simulink model "KaplunenkoDD_Task2"  (R2020a)
settings: Solver=VariableStepAuto  StartTime=0.0  StopTime=100  RelTol=1e-3  EnableMultiTasking=on
libraries: simulink x2
settings Model: Creator=Boris  LastModifiedBy=Dmitry Kaplunenko
settings DataIOCC: SaveOutput=off  SignalLogging=off  DSMLogging=off  SaveTime=off  ReturnWorkspaceOutputs=off
settings OptimizationCC: LifeSpan=inf
settings DebuggingCC: SFUnexpectedBacktrackingDiag=warning  SFNoUnconditionalDefaultTransitionDiag=warning  SFExecutionAtInitializationDiag=none  ArithmeticOperatorsInVariantConditions=warning
settings SFSimCC: SimUseLocalCustomCode=off  CustomCodeUndefinedFunction=UseInterfaceOnly
settings RTWCC: RTWUseLocalCustomCode=off
settings CodeAppCC: StateflowObjectComments=on
settings GRTTargetCC: TargetLangStandard=C89/C90 (ANSI)
settings ConfigComp: CovMetricSettings=dw  CovHtmlReporting=on  CovSaveCumulativeToWorkspaceVar=on  CovSaveSingleToWorkspaceVar=on  CovExternalEMLEnable=off

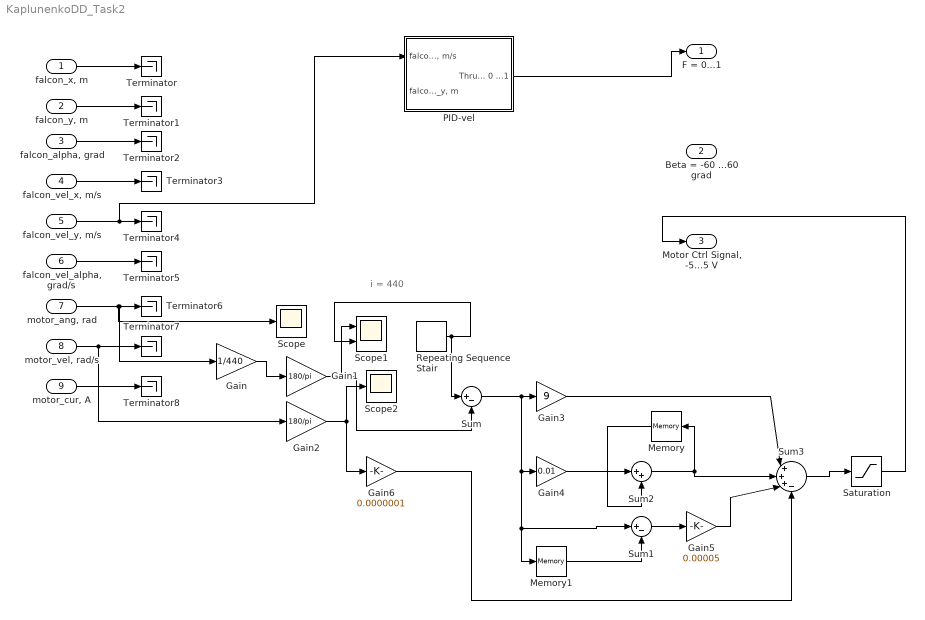
== system KaplunenkoDD_Task2 ==
  note: i = 440
  "falcon_x, m" : Inport  OutDataTypeStr=double  PortDimensions=1  SampleTime=[0.01,0]
  "falcon_y, m" : Inport  Port=2  OutDataTypeStr=double  PortDimensions=1  SampleTime=[0.01,0]
  "falcon_alpha, grad" : Inport  Port=3  OutDataTypeStr=double  PortDimensions=1  SampleTime=[0.01,0]
  "falcon_vel_x, m/s" : Inport  Port=4  OutDataTypeStr=double  PortDimensions=1  SampleTime=[0.01,0]
  "falcon_vel_y, m/s" : Inport  Port=5  OutDataTypeStr=double  PortDimensions=1  SampleTime=[0.01,0]
  "falcon_vel_alpha, grad/s" : Inport  Port=6  OutDataTypeStr=double  PortDimensions=1  SampleTime=[0.01,0]
  "motor_ang, rad" : Inport  Port=7  OutDataTypeStr=double  PortDimensions=1  SampleTime=[0.01,0]
  "motor_vel, rad/s" : Inport  Port=8  OutDataTypeStr=double  PortDimensions=1  SampleTime=[0.01,0]
  "motor_cur, A" : Inport  Port=9  OutDataTypeStr=double  PortDimensions=1  SampleTime=[0.01,0]
  Gain : Gain  Gain=1/440
  Gain1 : Gain  Gain=180/pi
  Gain2 : Gain  Gain=180/pi
  Gain3 : Gain  Gain=9
  Gain4 : Gain  Gain=0.01
  Gain5 : Gain  Gain=0.00005
  Gain6 : Gain  Gain=0.0000001
  Memory : Memory
  Memory1 : Memory
  PID-vel : Subsystem
  Repeating Sequence Stair : simulink/Sources/Repeating Sequence Stair  OutValues=[90 110 135].'  tsamp=15  OutMin=[]  OutMax=[]  OutDataTypeStr=double  OutputDataTypeScalingMode=double  OutDataType=fixdt(0,8)  ConRadixGroup=Best Precision: Vector-wise  OutScaling=2^-12
  Saturation : Saturate  UpperLimit=5  LowerLimit=-5
  Scope : Scope
  Scope1 : Scope  NumInputPorts=2
  Scope2 : Scope
  Sum : Sum  Inputs=|+-
  Sum1 : Sum  Inputs=|+-
  Sum2 : Sum  Inputs=|++
  Sum3 : Sum  Inputs=|+++-
  Terminator{,1..8} (9 alike) : Terminator
  F = 0...1 : Outport  OutDataTypeStr=double  PortDimensions=1  SampleTime=[0,1]  VectorParamsAs1DForOutWhenUnconnected=off
  Beta = -60 ...60 grad : Outport  Port=2  OutDataTypeStr=double  PortDimensions=1  VectorParamsAs1DForOutWhenUnconnected=off
  "Motor Ctrl Signal, -5...5 V" : Outport  Port=3  OutDataTypeStr=double  PortDimensions=1  SampleTime=[0,1]  VectorParamsAs1DForOutWhenUnconnected=off
  wires:
  "motor_ang, rad"/1 -> Scope/1, Terminator6/1, Gain/1
  "falcon_vel_y, m/s"/1 -> Terminator4/1, PID-vel/1("falcon_vel_Y, m/s")
  "falcon_vel_x, m/s"/1 -> Terminator3/1
  "falcon_alpha, grad"/1 -> Terminator2/1
  "falcon_y, m"/1 -> Terminator1/1
  "falcon_x, m"/1 -> Terminator/1
  "motor_vel, rad/s"/1 -> Terminator7/1, Gain2/1
  "motor_cur, A"/1 -> Terminator8/1
  "falcon_vel_alpha, grad/s"/1 -> Terminator5/1
  Gain/1 -> Gain1/1
  Gain1/1 -> Scope1/1, Sum/2
  Gain2/1 -> Scope2/1, Gain6/1
  Repeating Sequence Stair/1 -> Scope1/2, Sum/1
  Sum/1 -> Gain3/1, Gain4/1, Memory1/1, Sum1/1
  Gain4/1 -> Sum2/1
  Gain3/1 -> Sum3/1
  Sum2/1 -> Sum3/2, Memory/1
  Memory/1 -> Sum2/2
  Memory1/1 -> Sum1/2
  Sum1/1 -> Gain5/1
  Gain5/1 -> Sum3/3
  Sum3/1 -> Saturation/1
  Saturation/1 -> "Motor Ctrl Signal, -5...5 V"/1
  Gain6/1 -> Sum3/4
  PID-vel/1(Thrust = 0 ...1) -> F = 0...1/1

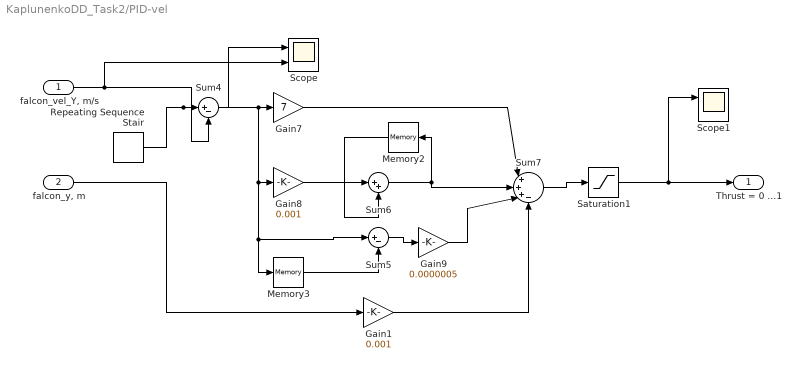
== system KaplunenkoDD_Task2/PID-vel ==
  "falcon_vel_Y, m/s" : Inport
  "falcon_y, m" : Inport  Port=2
  Gain1 : Gain  Gain=0.001
  Gain7 : Gain  Gain=7
  Gain8 : Gain  Gain=0.001
  Gain9 : Gain  Gain=0.0000005
  Memory2 : Memory
  Memory3 : Memory
  Repeating Sequence Stair : simulink/Sources/Repeating Sequence Stair  OutValues=[-20 -10 -5 -2.5 -1 ].'  tsamp=10  OutMin=[]  OutMax=[]  OutDataTypeStr=double  OutputDataTypeScalingMode=double  OutDataType=fixdt(0,8)  ConRadixGroup=Best Precision: Vector-wise  OutScaling=2^-12
  Saturation1 : Saturate  UpperLimit=1  LowerLimit=0
  Scope : Scope  NumInputPorts=2
  Scope1 : Scope  NumInputPorts=2
  Sum4 : Sum  Inputs=|+-
  Sum5 : Sum  Inputs=|+-
  Sum6 : Sum  Inputs=|++
  Sum7 : Sum  Inputs=|+++-
  Thrust = 0 ...1 : Outport
  wires:
  Repeating Sequence Stair/1 -> Sum4/1, Scope/1
  Gain9/1 -> Sum7/3
  Sum4/1 -> Sum5/1, Memory3/1, Gain8/1, Gain7/1
  Memory3/1 -> Sum5/2
  Gain8/1 -> Sum6/1
  Memory2/1 -> Sum6/2
  Gain7/1 -> Sum7/1
  Sum5/1 -> Gain9/1
  Sum6/1 -> Memory2/1, Sum7/2
  Sum7/1 -> Saturation1/1
  "falcon_vel_Y, m/s"/1 -> Scope/2, Sum4/2
  "falcon_y, m"/1 -> Gain1/1
  Saturation1/1 -> Scope1/1, Thrust = 0 ...1/1
  Gain1/1 -> Sum7/4
